simulink model "test_pos_ctrl_target"  (R2014a)
settings: Solver=ode5  StartTime=0.0  StopTime=inf  FixedStep=basic_time_step  RelTol=1e-3
values from neighbouring files (symbols this model uses):
  basic_time_step = 0.002    [init_pos_ctrl_target.m]
  g = 9.81    [init_pos_ctrl_target.m]
  kd = [2 0 0 ... (first row only)    [init_pos_ctrl_target.m]
  KDP = 11/5    (= 2.2)    [init_pos_ctrl_target.m]
  KDR = 11/5    (= 2.2)    [init_pos_ctrl_target.m]
  KDY = 11    [init_pos_ctrl_target.m]
  ki = 0*[.1 0 0 ... (first row only)    [init_pos_ctrl_target.m]
  kp = [1 0 0 ... (first row only)    [init_pos_ctrl_target.m]
  KPP = 30/5    (= 6)    [init_pos_ctrl_target.m]
  KPR = 30/5    (= 6)    [init_pos_ctrl_target.m]
  KPY = 30    [init_pos_ctrl_target.m]
  m0 = 1.3    [init_pos_ctrl_target.m]
  max_pitch = sin(15*pi/180)    [init_pos_ctrl_target.m]
  max_roll = sin(15*pi/180)    [init_pos_ctrl_target.m]
undefined symbols (not defined in the file or in its folder): DiscIntNeverNeededParam, IMU_time_step, n_robots, VICON_time_step
libraries: geometry_msgs x3, sensor_msgs x1, rt_sync x1
settings Model: Creator=prg  LastModifiedBy=fschiano
settings OptimizationCC: ExpressionDepthLimit=2147483647
settings DebuggingCC: UnderspecifiedInitializationDetection=Classic  StateNameClashWarn=warning

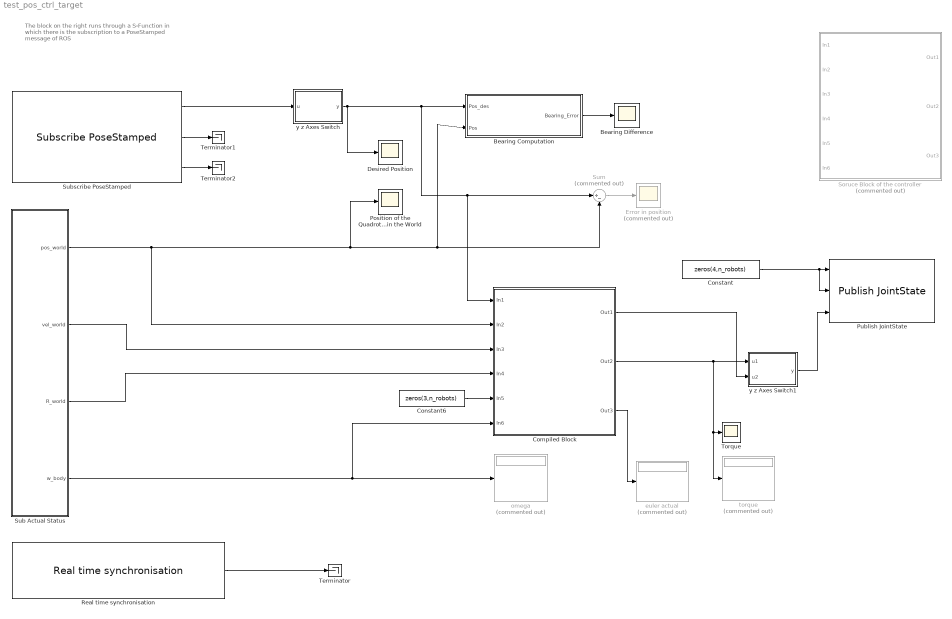
== system test_pos_ctrl_target ==
  note: The block on the right runs through a S-Function
      | in which there is the subscription to a PoseStamped
      | message of ROS
  Bearing Computation : Subsystem
  Bearing Difference : Scope
      settings: TimeRange=10000  YMin=-0.8  YMax=0.8  SaveName=ScopeData4
  Compiled Block : Subsystem
  Constant : Constant  Value=zeros(4,n_robots)  VectorParams1D=off
  Constant6 : Constant  Value=zeros(3,n_robots)
  Desired Position : Scope
      settings: TimeRange=10000  YMin=-4  YMax=7.5  SaveName=ScopeData3
  Error in position : Scope  Commented=on
      settings: TimeRange=10  YMin=-4  YMax=7.5
  "Position of the Quadrotor in the World " : Scope
      settings: TimeRange=10  YMin=-4  YMax=7.5  SaveName=ScopeData2
  Publish JointState : sensor_msgs/Publish JointState  stepTime=basic_time_step  topic_prefix='/command/quadrotor_'  list_of_robot_ids=char([0:n_robots-1])  topic_postfix=''  n_dofs=char(4)
  Real time synchronisation : rt_sync/Real time synchronisation  stepTime=basic_time_step  minShownDelay=0.5  ShowEveryNumCycles=1/basic_time_step  slowDownFactor=1
  Soruce Block of the controller : Subsystem  Commented=on
  Sub Actual Status : Subsystem
  Subscribe PoseStamped : geometry_msgs/Subscribe PoseStamped  stepTime=basic_time_step  topic_prefix='/vrep/Quadricopter_target_'  list_of_robot_ids=char([0:n_robots-1])  topic_postfix='/pose'
  Sum : Sum  Commented=on  Inputs=|+-
  Terminator : Terminator
  Terminator1 : Terminator
  Terminator2 : Terminator
  Torque : Scope
  euler actual : Display  Commented=on
  omega : Display  Commented=on
  "torque " : Display  Commented=on
  y z Axes Switch : MATLAB Function  TreatAsAtomicUnit=on
  y z Axes Switch1 : MATLAB Function  TreatAsAtomicUnit=on
  wires:
  Constant/1 -> Publish JointState/2, Publish JointState/1
  Sub Actual Status/4(w_body) -> Compiled Block/6(In6), omega/1
  Subscribe PoseStamped/1 -> y z Axes Switch/1(u)
  y z Axes Switch/1(y) -> Bearing Computation/1(Pos_des), Compiled Block/1(In1), Sum/1, Desired Position/1
  Sum/1 -> Error in position/1
  Real time synchronisation/1 -> Terminator/1
  Subscribe PoseStamped/2 -> Terminator1/1
  Subscribe PoseStamped/3 -> Terminator2/1
  Sub Actual Status/1(pos_world) -> Compiled Block/2(In2), Bearing Computation/2(Pos), Sum/2, "Position of the Quadrotor in the World "/1
  y z Axes Switch1/1(y) -> Publish JointState/3
  Compiled Block/2(Out2) -> "torque "/1, Torque/1, y z Axes Switch1/1(u1)
  Sub Actual Status/2(vel_world) -> Compiled Block/3(In3)
  Sub Actual Status/3("R_world ") -> Compiled Block/4(In4)
  Constant6/1 -> Compiled Block/5(In5)
  Compiled Block/1(Out1) -> y z Axes Switch1/2(u2)
  Compiled Block/3(Out3) -> euler actual/1
  Bearing Computation/1(Bearing_Error) -> Bearing Difference/1

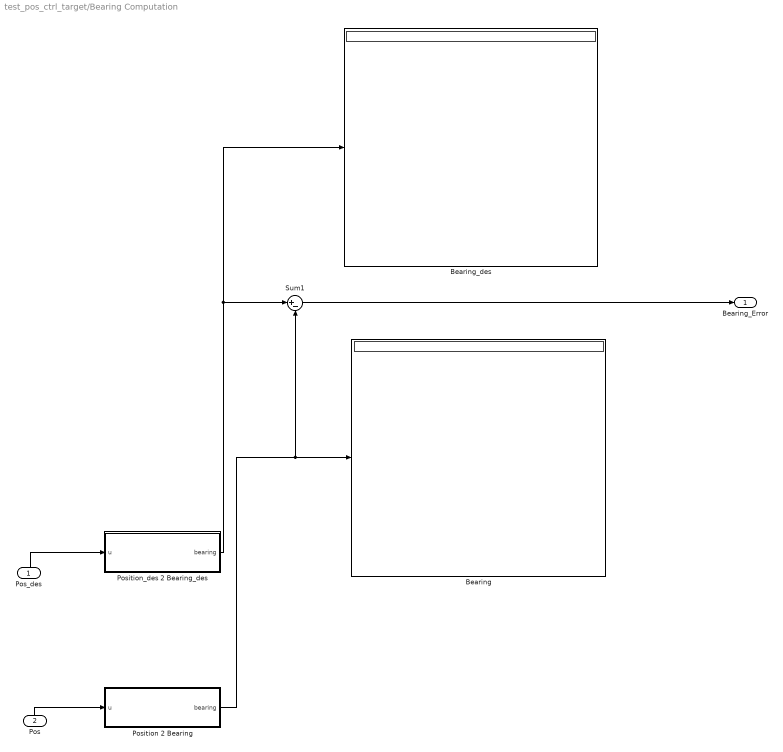
== system test_pos_ctrl_target/Bearing Computation ==
  Pos_des : Inport
  Pos : Inport  Port=2
  Bearing : Display
  "Bearing_des " : Display
  Position 2 Bearing : MATLAB Function  TreatAsAtomicUnit=on
  "Position_des 2 Bearing_des " : MATLAB Function  TreatAsAtomicUnit=on
  Sum1 : Sum  Inputs=|+-
  Bearing_Error : Outport
  wires:
  Pos/1 -> Position 2 Bearing/1(u)
  Pos_des/1 -> "Position_des 2 Bearing_des "/1(u)
  Position 2 Bearing/1(bearing) -> Bearing/1, Sum1/2
  Sum1/1 -> Bearing_Error/1
  "Position_des 2 Bearing_des "/1(bearing) -> Sum1/1, "Bearing_des "/1

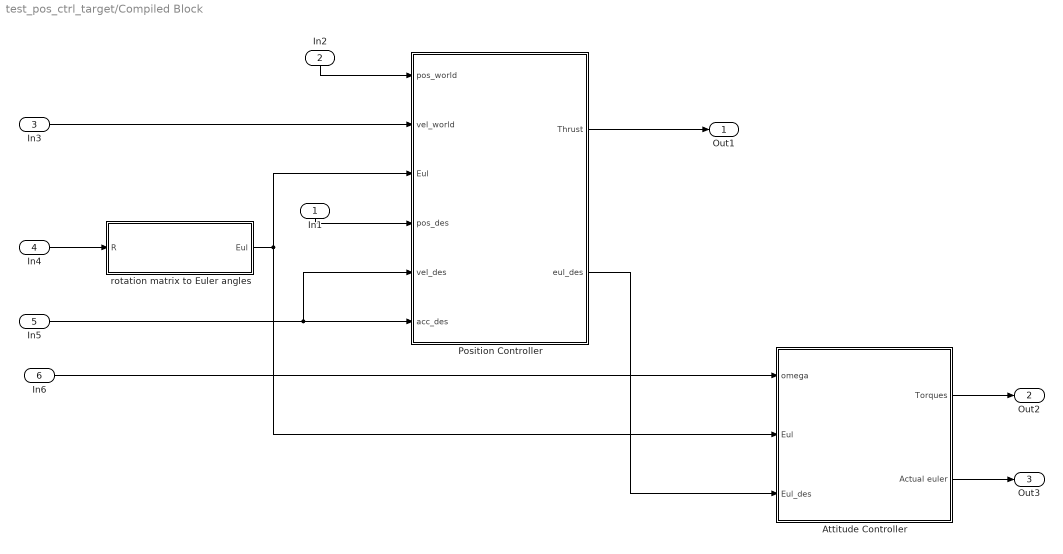
== system test_pos_ctrl_target/Compiled Block ==
  In1 : Inport
  In2 : Inport  Port=2
  In3 : Inport  Port=3
  In4 : Inport  Port=4
  In5 : Inport  Port=5
  In6 : Inport  Port=6
  Attitude Controller : Subsystem  SystemSampleTime=IMU_time_step
  Position Controller : Subsystem  SystemSampleTime=VICON_time_step
  rotation matrix to Euler angles : MATLAB Function  TreatAsAtomicUnit=on
  Out1 : Outport
  Out2 : Outport  Port=2
  Out3 : Outport  Port=3
  wires:
  In4/1 -> rotation matrix to Euler angles/1(R)
  rotation matrix to Euler angles/1(Eul) -> Attitude Controller/2(Eul), Position Controller/3(Eul)
  Attitude Controller/1(Torques) -> Out2/1
  In3/1 -> Position Controller/2(vel_world)
  In2/1 -> Position Controller/1(pos_world)
  Attitude Controller/2(Actual euler) -> Out3/1
  In1/1 -> Position Controller/4(pos_des)
  Position Controller/1(Thrust) -> Out1/1
  Position Controller/2(eul_des) -> Attitude Controller/3(Eul_des)
  In6/1 -> Attitude Controller/1(omega)
  In5/1 -> Position Controller/5(vel_des), Position Controller/6(acc_des)

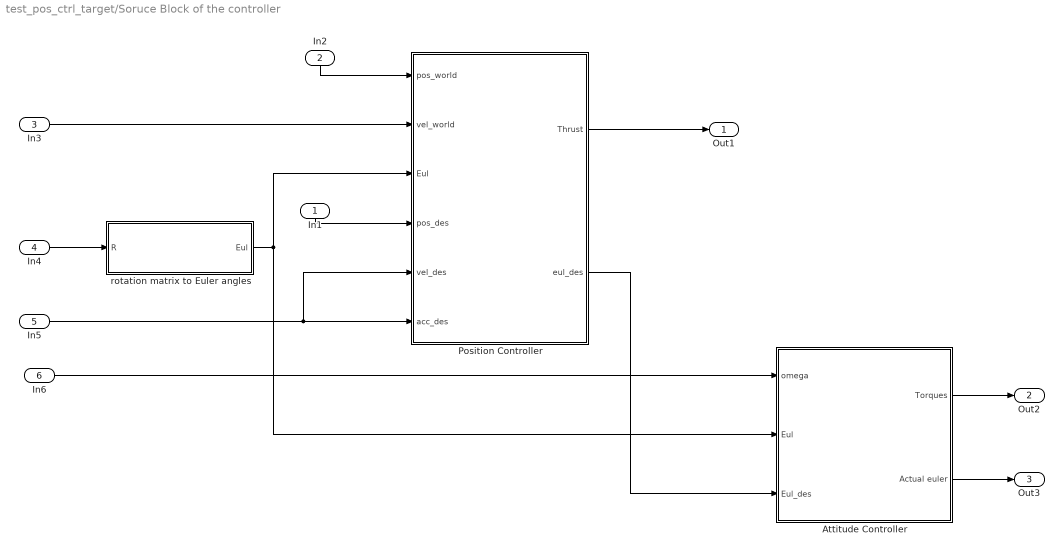
== system test_pos_ctrl_target/Soruce Block of the controller ==
  In1 : Inport
  In2 : Inport  Port=2
  In3 : Inport  Port=3
  In4 : Inport  Port=4
  In5 : Inport  Port=5
  In6 : Inport  Port=6
  Attitude Controller : Subsystem  SystemSampleTime=IMU_time_step
  Position Controller : Subsystem  SystemSampleTime=VICON_time_step
  rotation matrix to Euler angles : MATLAB Function  TreatAsAtomicUnit=on
  Out1 : Outport
  Out2 : Outport  Port=2
  Out3 : Outport  Port=3
  wires:
  In4/1 -> rotation matrix to Euler angles/1(R)
  rotation matrix to Euler angles/1(Eul) -> Attitude Controller/2(Eul), Position Controller/3(Eul)
  Attitude Controller/1(Torques) -> Out2/1
  In3/1 -> Position Controller/2(vel_world)
  In2/1 -> Position Controller/1(pos_world)
  Attitude Controller/2(Actual euler) -> Out3/1
  In1/1 -> Position Controller/4(pos_des)
  Position Controller/1(Thrust) -> Out1/1
  Position Controller/2(eul_des) -> Attitude Controller/3(Eul_des)
  In6/1 -> Attitude Controller/1(omega)
  In5/1 -> Position Controller/5(vel_des), Position Controller/6(acc_des)

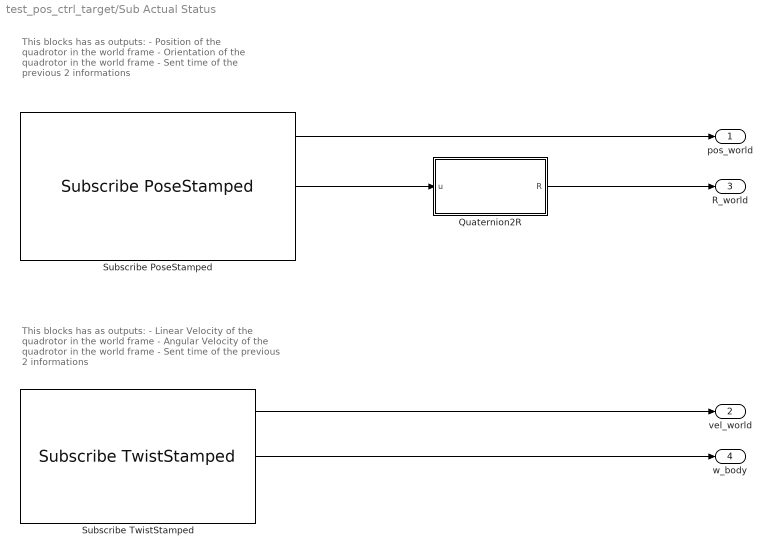
== system test_pos_ctrl_target/Sub Actual Status ==
  note: This blocks has as outputs:
      | - Linear Velocity of the quadrotor in the world frame
      | - Angular Velocity of the quadrotor in the world frame
      | - Sent time of the previous 2 informations
  note: This blocks has as outputs:
      | - Position of the quadrotor in the world frame
      | - Orientation of the quadrotor in the world frame
      | - Sent time of the previous 2 informations
  Quaternion2R : MATLAB Function  TreatAsAtomicUnit=on
  Subscribe PoseStamped : geometry_msgs/Subscribe PoseStamped  stepTime=basic_time_step  topic_prefix='/vrep/pose/quadrotor_'  list_of_robot_ids=char([0:n_robots-1])  topic_postfix=''
  Subscribe TwistStamped : geometry_msgs/Subscribe TwistStamped  stepTime=basic_time_step  topic_prefix='/vrep/twist/quadrotor_'  list_of_robot_ids=char([0:n_robots-1])  topic_postfix=''
  pos_world : Outport
  vel_world : Outport  Port=2
  "R_world " : Outport  Port=3
  w_body : Outport  Port=4
  wires:
  Subscribe PoseStamped/1 -> pos_world/1
  Subscribe PoseStamped/2 -> Quaternion2R/1(u)
  Quaternion2R/1(R) -> "R_world "/1
  Subscribe TwistStamped/1 -> vel_world/1
  Subscribe TwistStamped/2 -> w_body/1

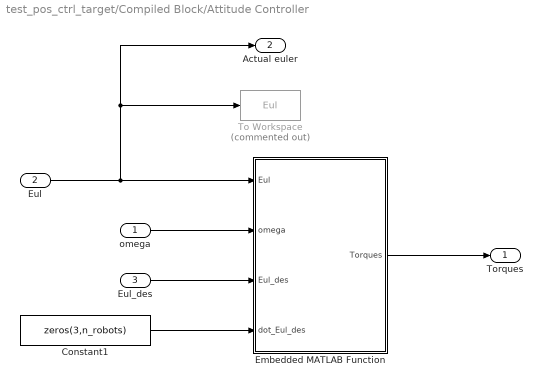
== system test_pos_ctrl_target/Compiled Block/Attitude Controller ==
  omega : Inport
  Eul : Inport  Port=2
  Eul_des : Inport  Port=3
  Constant1 : Constant  Value=zeros(3,n_robots)
  Embedded MATLAB Function : MATLAB Function  TreatAsAtomicUnit=on
  To Workspace : ToWorkspace  Commented=on  VariableName=Eul  SaveFormat=Structure With Time  SampleTime=-1
  Torques : Outport
  Actual euler : Outport  Port=2
  wires:
  Eul/1 -> Embedded MATLAB Function/1(Eul), Actual euler/1, To Workspace/1
  omega/1 -> Embedded MATLAB Function/2(omega)
  Eul_des/1 -> Embedded MATLAB Function/3(Eul_des)
  Embedded MATLAB Function/1(Torques) -> Torques/1
  Constant1/1 -> Embedded MATLAB Function/4(dot_Eul_des)

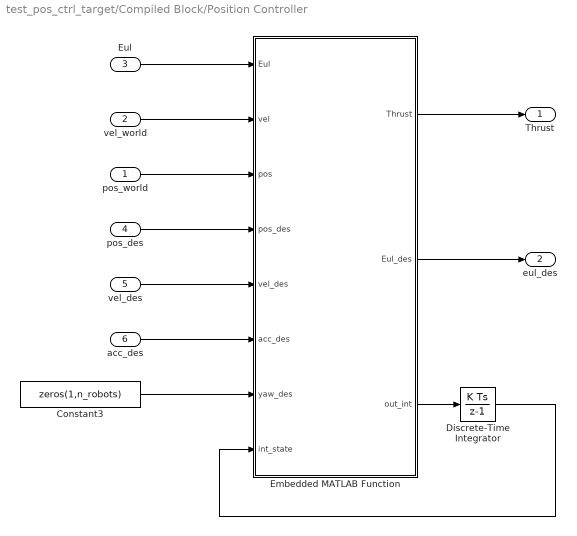
== system test_pos_ctrl_target/Compiled Block/Position Controller ==
  pos_world : Inport
  vel_world : Inport  Port=2
  Eul : Inport  Port=3
  pos_des : Inport  Port=4
  vel_des : Inport  Port=5
  acc_des : Inport  Port=6
  Constant3 : Constant  Value=zeros(1,n_robots)
  Discrete-Time Integrator : DiscreteIntegrator  InitialCondition=zeros(3,n_robots)  SampleTime=-1  OutDataTypeStr=Inherit: Inherit via back propagation  ICPrevOutput=DiscIntNeverNeededParam  ICPrevScaledInput=DiscIntNeverNeededParam
  Embedded MATLAB Function : MATLAB Function  TreatAsAtomicUnit=on
  Thrust : Outport
  eul_des : Outport  Port=2
  wires:
  Eul/1 -> Embedded MATLAB Function/1(Eul)
  vel_world/1 -> Embedded MATLAB Function/2(vel)
  pos_world/1 -> Embedded MATLAB Function/3(pos)
  Embedded MATLAB Function/1(Thrust) -> Thrust/1
  pos_des/1 -> Embedded MATLAB Function/4(pos_des)
  vel_des/1 -> Embedded MATLAB Function/5(vel_des)
  acc_des/1 -> Embedded MATLAB Function/6(acc_des)
  Constant3/1 -> Embedded MATLAB Function/7(yaw_des)
  Embedded MATLAB Function/3(out_int) -> Discrete-Time Integrator/1
  Discrete-Time Integrator/1 -> Embedded MATLAB Function/8(int_state)
  Embedded MATLAB Function/2(Eul_des) -> eul_des/1

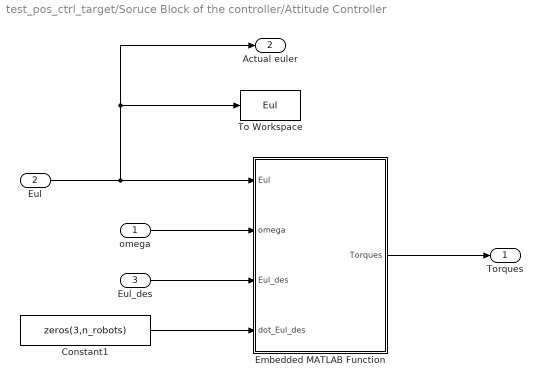
== system test_pos_ctrl_target/Soruce Block of the controller/Attitude Controller ==
  omega : Inport
  Eul : Inport  Port=2
  Eul_des : Inport  Port=3
  Constant1 : Constant  Value=zeros(3,n_robots)
  Embedded MATLAB Function : MATLAB Function  TreatAsAtomicUnit=on
  To Workspace : ToWorkspace  VariableName=Eul  SaveFormat=Structure With Time  SampleTime=-1
  Torques : Outport
  Actual euler : Outport  Port=2
  wires:
  Eul/1 -> Embedded MATLAB Function/1(Eul), Actual euler/1, To Workspace/1
  omega/1 -> Embedded MATLAB Function/2(omega)
  Eul_des/1 -> Embedded MATLAB Function/3(Eul_des)
  Embedded MATLAB Function/1(Torques) -> Torques/1
  Constant1/1 -> Embedded MATLAB Function/4(dot_Eul_des)

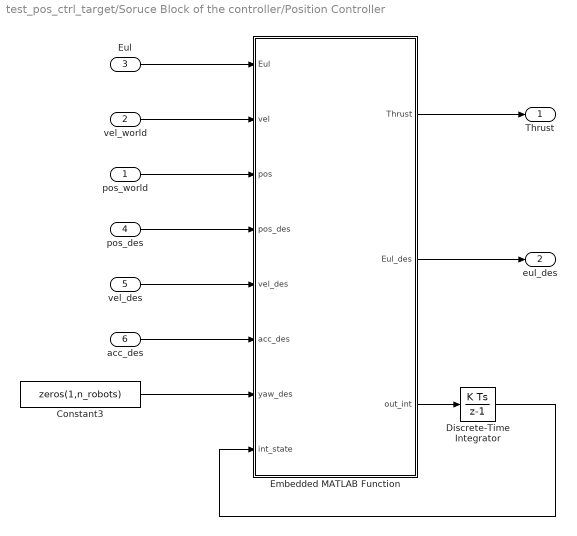
== system test_pos_ctrl_target/Soruce Block of the controller/Position Controller ==
  pos_world : Inport
  vel_world : Inport  Port=2
  Eul : Inport  Port=3
  pos_des : Inport  Port=4
  vel_des : Inport  Port=5
  acc_des : Inport  Port=6
  Constant3 : Constant  Value=zeros(1,n_robots)
  Discrete-Time Integrator : DiscreteIntegrator  InitialCondition=zeros(3,n_robots)  SampleTime=-1  OutDataTypeStr=Inherit: Inherit via back propagation  ICPrevOutput=DiscIntNeverNeededParam  ICPrevScaledInput=DiscIntNeverNeededParam
  Embedded MATLAB Function : MATLAB Function  TreatAsAtomicUnit=on
  Thrust : Outport
  eul_des : Outport  Port=2
  wires:
  Eul/1 -> Embedded MATLAB Function/1(Eul)
  vel_world/1 -> Embedded MATLAB Function/2(vel)
  pos_world/1 -> Embedded MATLAB Function/3(pos)
  Embedded MATLAB Function/1(Thrust) -> Thrust/1
  pos_des/1 -> Embedded MATLAB Function/4(pos_des)
  vel_des/1 -> Embedded MATLAB Function/5(vel_des)
  acc_des/1 -> Embedded MATLAB Function/6(acc_des)
  Constant3/1 -> Embedded MATLAB Function/7(yaw_des)
  Embedded MATLAB Function/3(out_int) -> Discrete-Time Integrator/1
  Discrete-Time Integrator/1 -> Embedded MATLAB Function/8(int_state)
  Embedded MATLAB Function/2(Eul_des) -> eul_des/1

== matlab function test_pos_ctrl_target/Soruce Block of the controller/Attitude Controller/Embedded MATLAB Function ==
  data: Eul input size=3,n_robots; Torques output size=3,n_robots; omega input size=3,n_robots; Eul_des input size=3,n_robots; dot_Eul_des input size=3,n_robots; KDR parameter; KPR parameter; KDP parameter; KPP parameter; KDY parameter; KPY parameter; n_robots parameter
% OLD FUNCTION (without parametrization for n_robots)
function Torques  = fcn(Eul, omega, Eul_des, dot_Eul_des, KDR, KPR, KDP, KPP, KDY, KPY, n_robots)
% This block supports the Embedded MATLAB subset.
% See the help menu for details.

% p = angles(2);
% r = angles(1);
% y=angles(3);
%
% T = [1      tan(p)*sin(r) tan(p)*cos(r);
%     0       cos(r)  -sin(r);
%     0       sin(r)/cos(p)   cos(r)/cos(p)];
%
% dot_ang = T*omega;
% dot_r=dot_ang(1);
% dot_p = dot_ang(2);
%
% T_dot = [0  tan(p)*cos(r)*dot_r+(sin(r)+tan(p)^2*sin(r))*dot_p -tan(p)*sin(r)*dot_r+(cos(r)+tan(p)^2*cos(r))*dot_p;
%          0  -sin(r)*dot_r   -cos(r)*dot_r;
%          0  cos(r)/cos(p)*dot_r+sin(r)*sin(p)/cos(p)^2*dot_p    -sin(r)/cos(p)*dot_r+cos(r)*sin(p)/cos(p)^2*dot_p];
%
%
% k_d = 11;
% k_p = 30;
% ang_vel_des = [0 0 yaw_dot_des]';
%
%
% if(yaw_des - angles(3) > pi)
%     angles(3) = angles(3)+2*pi;
% elseif (yaw_des - angles(3) < -pi)
%     angles(3) = angles(3)-2*pi;
% end
%
% ang_des = [roll_des pitch_des yaw_des]';
% U = I*inv(T)*(k_d*(ang_vel_des-dot_ang)+k_p*(ang_des - angles)-T_dot*omega)+cross(omega, I*omega);
% r_c = U(1);
% p_c = U(2);
% y_c = U(3);

Torques=[zeros(1,n_robots);zeros(1,n_robots);zeros(1,n_robots)];

% Extract Roll pitch and yaw angles w.r.t. the i-th robot
r = reshape(Eul(1,:),[1,1,n_robots]);
p = reshape(Eul(2,:),[1,1,n_robots]);
y = reshape(Eul(3,:),[1,1,n_robots]);

T = [ones(1,1,n_robots)       tan(p).*sin(r)  tan(p).*cos(r);
     zeros(1,1,n_robots)      cos(r)         -sin(r);
     zeros(1,1,n_robots)      sin(r)./cos(p)  cos(r)./cos(p)];


% T=eye(3);

dot_Eul = zeros(3,n_robots);

for i=1:n_robots
    dot_Eul(:,i)=reshape(T(:,:,i),[3,3])*omega(:,i);
end

% dot_Eul = T*omega;

dot_r = dot_Eul(1,:);
dot_p = dot_Eul(2,:);
dot_y = dot_Eul(3,:);

% U=I*inv(T)*([ KDR * (0 - dot_r) + KPR * (roll_des - r); KDP * (0 - dot_p) + KPP * (pitch_des - p) ; KPY * (yaw_dot_des - dot_y) ]);

r = reshape(r,[1,n_robots]);
p = reshape(p,[1,n_robots]);
y = reshape(y,[1,n_robots]);

Torques(1,:) = KDR * (dot_Eul_des(1,:) - dot_r) + KPR * (Eul_des(1,:) - r);
Torques(2,:) = KDP * (dot_Eul_des(2,:) - dot_p) + KPP * (Eul_des(2,:) - p);
Torques(3,:) = KDY * (dot_Eul_des(3,:) - dot_y) + KPY * (Eul_des(3,:) - y);


% if abs(Torques(1)) > 0.02
%     Torques(1)= 0.02;
%
% end
%
%
% if abs(Torques(2)) > 0.02
%     Torques(2)= 0.02;
%
% end

== matlab function test_pos_ctrl_target/Sub Actual Status/Quaternion2R ==
  data: u input size=4,n_robots; R output size=n_robots,3,3; n_robots parameter
function R = fcn(u, n_robots)

w = u(1,:);
x = u(2,:);
y = u(3,:);
z = u(4,:);

n = sqrt(x.*x + y.*y + z.*z + w.*w);

x = x./n;
y = y./n;
z = z./n;
w = w./n;

Rxx = reshape(1 - 2*(y.^2 + z.^2),[1,1,n_robots]);
Rxy = reshape(2*(x.*y - z.*w),[1,1,n_robots]);
Rxz = reshape(2*(x.*z + y.*w),[1,1,n_robots]);

Ryx = reshape(2*(x.*y + z.*w),[1,1,n_robots]);
Ryy = reshape(1 - 2*(x.^2 + z.^2),[1,1,n_robots]);
Ryz = reshape(2*(y.*z - x.*w ),[1,1,n_robots]);

Rzx = reshape(2*(x.*z - y.*w ),[1,1,n_robots]);
Rzy = reshape(2*(y.*z + x.*w ),[1,1,n_robots]);
Rzz = reshape(1 - 2 *(x.^2 + y.^2),[1,1,n_robots]);

R_temp = [
    Rxx,    Rxy,    Rxz;
    Ryx,    Ryy,    Ryz;
    Rzx,    Rzy,    Rzz;];

% R_temp = [
%     Rxx,    Ryx,    Rzx;
%     Rxy,    Ryy,    Rzy;
%     Rxz,    Ryz,    Rzz;];

% for i=1:n_robots
%     R_temp(:,:,i)=R_temp(:,:,i)';
% end

R=reshape(R_temp,n_robots,3,3);
% R=rand(1,3,3);

% a = u( 1 );
% b = u( 2 );
% c = u( 3 );
% d = u( 4 );
%
%
%   R(1,1) = a*a+b*b-c*c-d*d;
%   R(1,2) = 2*b*c-2*a*d;
%   R(1,3) = 2*a*c+2*b*d;
%
%   R(2,1)   = 2*a*d+2*b*c;
%   R(2,2)  = a*a-b*b+c*c-d*d;
%   R(2,3)  = 2*c*d-2*a*b;
%
%   R(3,1)    = 2*b*d-2*a*c;
%   R(3,2)    = 2*a*b+2*c*d;
%   R(3,3)    = a*a-b*b-c*c+d*d;


% % VERSION WITH THE FOR CYCLE
%
%
% % u is the vector of the quaternions.
% % If there are 2 robots involved the u will look like this:
% % u=[w1 x1 y1 z1 w2 x2 y2 z2]'
%
% %#codegen
% assert(n_robots<40);
%
% % Initialization of the variables. If you remove this it won't work because
% % code generation doesn't support dynamic changing size variables.
% w=zeros(n_robots,1);
% x=zeros(n_robots,1);
% y=zeros(n_robots,1);
% z=zeros(n_robots,1);
% n=zeros(n_robots,1);
%
% Rxx=zeros(n_robots,1);
% Rxy=zeros(n_robots,1);
% Rxz=zeros(n_robots,1);
% Ryx=zeros(n_robots,1);
% Ryy=zeros(n_robots,1);
% Ryz=zeros(n_robots,1);
% Rzx=zeros(n_robots,1);
% Rzy=zeros(n_robots,1);
% Rzz=zeros(n_robots,1);
%
% R=zeros(3*n_robots,3);
%
% for i=0:n_robots-1
%
%     w(i+1) = u( 1+3*i );
%     x(i+1) = u( 2+3*i );
%     y(i+1) = u( 3+3*i );
%     z(i+1) = u( 4+3*i );
%
%     n(i+1) = sqrt(x(i+1)*x(i+1) + y(i+1)*y(i+1) + z(i+1)*z(i+1) + w(i+1)*w(i+1));
%
%     x(i+1) = x(i+1)/ n(i+1);
%     y(i+1) = y(i+1)/ n(i+1);
%     z(i+1) = z(i+1)/ n(i+1);
%     w(i+1) = w(i+1)/ n(i+1);
%
%     Rxx(i+1) = 1 - 2*(y(i+1)^2 + z(i+1)^2);
%     Rxy(i+1) = 2*(x(i+1)*y(i+1) - z(i+1)*w(i+1));
%     Rxz(i+1) = 2*(x(i+1)*z(i+1) + y(i+1)*w(i+1));
%
%     Ryx(i+1) = 2*(x(i+1)*y(i+1) + z(i+1)*w(i+1));
%     Ryy(i+1) = 1 - 2*(x(i+1)^2 + z(i+1)^2);
%     Ryz(i+1) = 2*(y(i+1)*z(i+1) - x(i+1)*w(i+1) );
%
%     Rzx(i+1) = 2*(x(i+1)*z(i+1) - y(i+1)*w(i+1) );
%     Rzy(i+1) = 2*(y(i+1)*z(i+1) + x(i+1)*w(i+1) );
%     Rzz(i+1) = 1 - 2 *(x(i+1)^2 + y(i+1)^2);
%
%     R((1+i*3):(3+i*3),:) = [
%         Rxx(i+1),    Rxy(i+1),    Rxz(i+1);
%         Ryx(i+1),    Ryy(i+1),    Ryz(i+1);
%         Rzx(i+1),    Rzy(i+1),    Rzz(i+1)];
%
%     %     R_vectorized=R(:);
% end

== matlab function test_pos_ctrl_target/Soruce Block of the controller/Position Controller/Embedded MATLAB Function ==
  data: Eul input size=3,n_robots; Thrust output size=1,n_robots; Eul_des output size=3,n_robots; vel input size=3,n_robots; pos input size=3,n_robots; pos_des input size=3,n_robots; vel_des input size=3,n_robots; acc_des input size=3,n_robots; yaw_des input size=1,n_robots; int_state input size=3,n_robots; m0 parameter; g parameter; out_int output size=3,n_robots; kd parameter; kp parameter; ki parameter; max_roll parameter; max_pitch parameter; n_robots parameter
% Before the function was like that:
% function [Thrust, roll_des, pitch_des, yaw_dot_des, out_int]  = fcn(Eul, vel, pos, pos_des, vel_des, acc_des, yaw_des, int_state, m0, g, kd, kp, ki, max_roll, max_pitch,n_robots)

% Now I fused 3 variables roll_des, pitch_des, yaw_dot_des into Eul_des
function [Thrust, Eul_des, out_int]  = fcn(Eul, vel, pos, pos_des, vel_des, acc_des, yaw_des, int_state, m0, g, kd, kp, ki, max_roll, max_pitch,n_robots)
% This block supports the Embedded MATLAB subset
% See the help menu for details.

% Definition of the variables. For code generation, the first appearance
% of a variable must establish its size. The first appearance of a variable
% cannot be subscripted.

% r=zeros(n_robots,1);
% p=zeros(n_robots,1);
% y=zeros(n_robots,1);

% Thrust=zeros(n_robots,1);
%
% ddpx=zeros(n_robots,1);
% ddpy=zeros(n_robots,1);
%
% ctrl_roll=zeros(n_robots,1);
% ctrl_pitch=zeros(n_robots,1);
%
% roll_des=zeros(n_robots,1);
% pitch_des=zeros(n_robots,1);
% yaw_dot_des=zeros(n_robots,1);

% Extract Roll pitch and yaw angles w.r.t. the i-th robot
r = Eul(1,:);
p = Eul(2,:);
y = Eul(3,:);

% term_1=m0./(cos(r).*cos(p));
% term_2=(-g + acc_des(3,:) + kd(3,3)*(vel_des(3,:)-vel(3,:)) + kp(3,3)*(pos_des(3,:)-pos(3,:)) + int_state(3,:));
% term_3=term_1*term_2;

% Compute the Thrust w.r.t. the i-th robot
Thrust=m0./(cos(r).*cos(p)).*(-g + acc_des(3,:) + kd(3,3)*(vel_des(3,:)-vel(3,:)) + kp(3,3)*(pos_des(3,:)-pos(3,:)) + int_state(3,:) );

out_int=ki*(pos_des-pos);

% Saturation of the Thrust

for i=1:n_robots
    if (Thrust(1,i)>-5)
        Thrust(1,i)=-5;
    end
end

% max_T=30;
%
% if abs(T(3))>max_T
%     T(3)=sign(T(3))*max_T;
% end

% Thrust needed to hover ???
for i=1:n_robots
    if (Thrust(1,i)<-2*m0*g+5)
        Thrust(1,i)=-2*m0*g+5;
    end
end

% roll_des=-m/T(3)*( acc_des(2) + kd*(vel_des(2) -vel(2)) + kp*(pos_des(2)-pos(2)) );
% pitch_des=m/T(3)*( acc_des(1) + kd*(vel_des(1) -vel(1)) + kp*(pos_des(1)-pos(1)) );

ddpx=kd(1,1)*(vel_des(1,:) -vel(1,:)) + kp(1,1)*(pos_des(1,:)-pos(1,:) + int_state(1,:) );
ddpy=kd(2,2)*(vel_des(2,:) -vel(2,:)) + kp(2,2)*(pos_des(2,:)-pos(2,:) + int_state(2,:) );

ctrl_roll=m0./Thrust.*( -sin(y).*ddpx+cos(y).*ddpy);

% Saturation of the roll_ctrl
for i=1:n_robots
    if abs(ctrl_roll(1,i))>max_roll
        ctrl_roll(1,i)=sign(ctrl_roll(1,i))*max_roll;
    end 
end

ctrl_pitch= m0./(Thrust.*cos(r)).*( cos(y).*ddpx+sin(y).*ddpy);

% Saturation of the pitch_ctrl
for i=1:n_robots
    if abs(ctrl_pitch(1,i))>max_pitch
        ctrl_pitch(1,i)=sign(ctrl_pitch(1,i))*max_pitch;
    end
end


roll_des = -asin( ctrl_roll );

pitch_des = asin(  ctrl_pitch );

yaw_dot_des = zeros(1,n_robots); % kp(3,3)*(yaw_des-y);

Eul_des=([roll_des;pitch_des; yaw_dot_des]);


%% OLD FUNCTION (not parametrized for n_robots)
% function [Thrust, roll_des, pitch_des, yaw_dot_des, out_int]  = fcn(Eul, vel, pos, pos_des, vel_des, acc_des, yaw_des, int_state, m0, g, kd, kp, ki, max_roll, max_pitch)
% % This block supports the Embedded MATLAB subset
% % See the help menu for details.
%
%
% r = Eul(1);
% p = Eul(2);
% y = Eul(3);
%
%
%
% Thrust=m0/(cos(r)*cos(p))*(-g + acc_des(3) + kd(3,3)*(vel_des(3) -vel(3)) + kp(3,3)*(pos_des(3)-pos(3)) + int_state(3) );
%
%
% out_int=ki*(pos_des-pos);
%
%
%
% % max_T=30;
% %
% % if abs(T(3))>max_T
% %     T(3)=sign(T(3))*max_T;
% % end
%
% if (Thrust>-5)
%     Thrust=-5;
% end
%
%
% if (Thrust<-2*m0*g+5)
%     Thrust=-2*m0*g+5;
% end
%
%
%
%
% % roll_des=-m/T(3)*( acc_des(2) + kd*(vel_des(2) -vel(2)) + kp*(pos_des(2)-pos(2)) );
% % pitch_des=m/T(3)*( acc_des(1) + kd*(vel_des(1) -vel(1)) + kp*(pos_des(1)-pos(1)) );
%
%
% ddpx=kd(1,1)*(vel_des(1) -vel(1)) + kp(1,1)*(pos_des(1)-pos(1) + int_state(1) );
% ddpy=kd(2,2)*(vel_des(2) -vel(2)) + kp(2,2)*(pos_des(2)-pos(2) + int_state(2) );
%
%
%
% ctrl_roll=m0/Thrust*( -sin(y)*ddpx+cos(y)*ddpy);
%
% if abs(ctrl_roll)>max_roll
%     ctrl_roll=sign(ctrl_roll)*max_roll;
% end
%
% ctrl_pitch= m0/(Thrust*cos(r))*( cos(y)*ddpx+sin(y)*ddpy);
%
%
% if abs(ctrl_pitch)>max_pitch
%     ctrl_pitch=sign(ctrl_pitch)*max_pitch;
% end
%
%
%
%
%
% roll_des = -asin( ctrl_roll );
%
% pitch_des = asin(  ctrl_pitch );
%
% yaw_dot_des = 0; % kp(3,3)*(yaw_des-y);

== matlab function test_pos_ctrl_target/Soruce Block of the controller/rotation matrix to Euler angles ==
  data: R input size=n_robots,3,3 [..10]; Eul output size=3,n_robots; n_robots parameter
function Eul = eulerangles(R, n_robots)
% This block supports an embeddable subset of the MATLAB language.
% See the help menu for details.

R=reshape(R,[3,3,n_robots]);

Roll = atan2(R(3,2,:),R(3,3,:));
Pitch = atan2(-R(3,1,:),sqrt(R(3,2,:).^2+R(3,3,:).^2));
Yaw = atan2(R(2,1,:),R(1,1,:));

% From the previous instructions if R is a 3D matrix of 3 x 3 x n_robots I
% will have Roll Pitch and Yaw which will be 3 3D matrix with dimensions 1
% x 1 x n_robots. For this reason I need a reshape which will give
% transform Roll, Pitch and Yaw in vectors with dimensions 1 x n_robots

Roll = reshape(Roll,1,n_robots);
Pitch = reshape(Pitch,1,n_robots);
Yaw = reshape(Yaw,1,n_robots);

% The following Eul variable will be a 3 x n_robots matrix
Eul = [Roll; Pitch; Yaw];


% function Eul = eulerangles(R,n_robots)
% % This block supports an embeddable subset of the MATLAB language.
% % See the help menu for details.
% 
% % R=reshape(R_vectorized,[3,3,n_robots]);
% 
% Roll=zeros(n_robots);
% Pitch=zeros(n_robots);
% Yaw=zeros(n_robots);
% Eul=zeros(n_robots,3);
% 
% for i=1:n_robots
%     
%     Roll(i) = atan2(R(3+(n_robots-1)*3,2,i),R(3+(n_robots-1)*3,3,i));
%     Pitch(i) = atan2(-R(3+(n_robots-1)*3,1,i),sqrt(R(3+(n_robots-1)*3,2,i)^2+R(3+(n_robots-1)*3,3,i)^2));
%     Yaw(i) = atan2(R(2+(n_robots-1)*3,1,i),R(1+(n_robots-1)*3,1,i));
%     
%     Eul(i) = [Roll(i) Pitch(i) Yaw(i)];
% end

== matlab function test_pos_ctrl_target/Compiled Block/Attitude Controller/Embedded MATLAB Function ==
  data: Eul input size=3,n_robots; Torques output size=3,n_robots; omega input size=3,n_robots; Eul_des input size=3,n_robots; dot_Eul_des input size=3,n_robots; KDR parameter; KPR parameter; KDP parameter; KPP parameter; KDY parameter; KPY parameter; n_robots parameter
% OLD FUNCTION (without parametrization for n_robots)
function Torques  = fcn(Eul, omega, Eul_des, dot_Eul_des, KDR, KPR, KDP, KPP, KDY, KPY, n_robots)
% This block supports the Embedded MATLAB subset.
% See the help menu for details.

% p = angles(2);
% r = angles(1);
% y=angles(3);
%
% T = [1      tan(p)*sin(r) tan(p)*cos(r);
%     0       cos(r)  -sin(r);
%     0       sin(r)/cos(p)   cos(r)/cos(p)];
%
% dot_ang = T*omega;
% dot_r=dot_ang(1);
% dot_p = dot_ang(2);
%
% T_dot = [0  tan(p)*cos(r)*dot_r+(sin(r)+tan(p)^2*sin(r))*dot_p -tan(p)*sin(r)*dot_r+(cos(r)+tan(p)^2*cos(r))*dot_p;
%          0  -sin(r)*dot_r   -cos(r)*dot_r;
%          0  cos(r)/cos(p)*dot_r+sin(r)*sin(p)/cos(p)^2*dot_p    -sin(r)/cos(p)*dot_r+cos(r)*sin(p)/cos(p)^2*dot_p];
%
%
% k_d = 11;
% k_p = 30;
% ang_vel_des = [0 0 yaw_dot_des]';
%
%
% if(yaw_des - angles(3) > pi)
%     angles(3) = angles(3)+2*pi;
% elseif (yaw_des - angles(3) < -pi)
%     angles(3) = angles(3)-2*pi;
% end
%
% ang_des = [roll_des pitch_des yaw_des]';
% U = I*inv(T)*(k_d*(ang_vel_des-dot_ang)+k_p*(ang_des - angles)-T_dot*omega)+cross(omega, I*omega);
% r_c = U(1);
% p_c = U(2);
% y_c = U(3);

Torques=[zeros(1,n_robots);zeros(1,n_robots);zeros(1,n_robots)];

% Extract Roll pitch and yaw angles w.r.t. the i-th robot
r = reshape(Eul(1,:),[1,1,n_robots]);
p = reshape(Eul(2,:),[1,1,n_robots]);
y = reshape(Eul(3,:),[1,1,n_robots]);

T = [ones(1,1,n_robots)       tan(p).*sin(r)  tan(p).*cos(r);
     zeros(1,1,n_robots)      cos(r)         -sin(r);
     zeros(1,1,n_robots)      sin(r)./cos(p)  cos(r)./cos(p)];


% T=eye(3);

dot_Eul = zeros(3,n_robots);

for i=1:n_robots
    dot_Eul(:,i)=reshape(T(:,:,i),[3,3])*omega(:,i);
end

% dot_Eul = T*omega;

dot_r = dot_Eul(1,:);
dot_p = dot_Eul(2,:);
dot_y = dot_Eul(3,:);

% U=I*inv(T)*([ KDR * (0 - dot_r) + KPR * (roll_des - r); KDP * (0 - dot_p) + KPP * (pitch_des - p) ; KPY * (yaw_dot_des - dot_y) ]);

r = reshape(r,[1,n_robots]);
p = reshape(p,[1,n_robots]);
y = reshape(y,[1,n_robots]);

Torques(1,:) = KDR * (dot_Eul_des(1,:) - dot_r) + KPR * (Eul_des(1,:) - r);
Torques(2,:) = KDP * (dot_Eul_des(2,:) - dot_p) + KPP * (Eul_des(2,:) - p);
Torques(3,:) = KDY * (dot_Eul_des(3,:) - dot_y) + KPY * (Eul_des(3,:) - y);


% if abs(Torques(1)) > 0.02
%     Torques(1)= 0.02;
%
% end
%
%
% if abs(Torques(2)) > 0.02
%     Torques(2)= 0.02;
%
% end

== matlab function test_pos_ctrl_target/y z Axes Switch ==
  data: u input size=3,n_robots; y output size=3,n_robots; n_robots parameter
function y = fcn(u, n_robots)

y=[u(1,:);-u(2,:);-u(3,:)];

end

== matlab function test_pos_ctrl_target/y z Axes Switch1 ==
  data: u1 input; u2 input; y output; n_robots parameter
function y = fcn(u1,u2, n_robots)

y=[u1;u2];

end

== matlab function test_pos_ctrl_target/Compiled Block/Position Controller/Embedded MATLAB Function ==
  data: Eul input size=3,n_robots; Thrust output size=1,n_robots; Eul_des output size=3,n_robots; vel input size=3,n_robots; pos input size=3,n_robots; pos_des input size=3,n_robots; vel_des input size=3,n_robots; acc_des input size=3,n_robots; yaw_des input size=1,n_robots; int_state input size=3,n_robots; m0 parameter; g parameter; out_int output size=3,n_robots; kd parameter; kp parameter; ki parameter; max_roll parameter; max_pitch parameter; n_robots parameter
% Before the function was like that:
% function [Thrust, roll_des, pitch_des, yaw_dot_des, out_int]  = fcn(Eul, vel, pos, pos_des, vel_des, acc_des, yaw_des, int_state, m0, g, kd, kp, ki, max_roll, max_pitch,n_robots)

% Now I fused 3 variables roll_des, pitch_des, yaw_dot_des into Eul_des
function [Thrust, Eul_des, out_int]  = fcn(Eul, vel, pos, pos_des, vel_des, acc_des, yaw_des, int_state, m0, g, kd, kp, ki, max_roll, max_pitch,n_robots)
% This block supports the Embedded MATLAB subset
% See the help menu for details.

% Definition of the variables. For code generation, the first appearance
% of a variable must establish its size. The first appearance of a variable
% cannot be subscripted.

% r=zeros(n_robots,1);
% p=zeros(n_robots,1);
% y=zeros(n_robots,1);

% Thrust=zeros(n_robots,1);
%
% ddpx=zeros(n_robots,1);
% ddpy=zeros(n_robots,1);
%
% ctrl_roll=zeros(n_robots,1);
% ctrl_pitch=zeros(n_robots,1);
%
% roll_des=zeros(n_robots,1);
% pitch_des=zeros(n_robots,1);
% yaw_dot_des=zeros(n_robots,1);

% Extract Roll pitch and yaw angles w.r.t. the i-th robot
r = Eul(1,:);
p = Eul(2,:);
y = Eul(3,:);

% term_1=m0./(cos(r).*cos(p));
% term_2=(-g + acc_des(3,:) + kd(3,3)*(vel_des(3,:)-vel(3,:)) + kp(3,3)*(pos_des(3,:)-pos(3,:)) + int_state(3,:));
% term_3=term_1*term_2;

% Compute the Thrust w.r.t. the i-th robot
Thrust=m0./(cos(r).*cos(p)).*(-g + acc_des(3,:) + kd(3,3)*(vel_des(3,:)-vel(3,:)) + kp(3,3)*(pos_des(3,:)-pos(3,:)) + int_state(3,:) );

out_int=ki*(pos_des-pos);

% Saturation of the Thrust

for i=1:n_robots
    if (Thrust(1,i)>-5)
        Thrust(1,i)=-5;
    end
end

% max_T=30;
%
% if abs(T(3))>max_T
%     T(3)=sign(T(3))*max_T;
% end

% Thrust needed to hover ???
for i=1:n_robots
    if (Thrust(1,i)<-2*m0*g+5)
        Thrust(1,i)=-2*m0*g+5;
    end
end

% roll_des=-m/T(3)*( acc_des(2) + kd*(vel_des(2) -vel(2)) + kp*(pos_des(2)-pos(2)) );
% pitch_des=m/T(3)*( acc_des(1) + kd*(vel_des(1) -vel(1)) + kp*(pos_des(1)-pos(1)) );

ddpx=kd(1,1)*(vel_des(1,:) -vel(1,:)) + kp(1,1)*(pos_des(1,:)-pos(1,:) + int_state(1,:) );
ddpy=kd(2,2)*(vel_des(2,:) -vel(2,:)) + kp(2,2)*(pos_des(2,:)-pos(2,:) + int_state(2,:) );

ctrl_roll=m0./Thrust.*( -sin(y).*ddpx+cos(y).*ddpy);

% Saturation of the roll_ctrl
for i=1:n_robots
    if abs(ctrl_roll(1,i))>max_roll
        ctrl_roll(1,i)=sign(ctrl_roll(1,i))*max_roll;
    end 
end

ctrl_pitch= m0./(Thrust.*cos(r)).*( cos(y).*ddpx+sin(y).*ddpy);

% Saturation of the pitch_ctrl
for i=1:n_robots
    if abs(ctrl_pitch(1,i))>max_pitch
        ctrl_pitch(1,i)=sign(ctrl_pitch(1,i))*max_pitch;
    end
end


roll_des = -asin( ctrl_roll );

pitch_des = asin(  ctrl_pitch );

yaw_dot_des = zeros(1,n_robots); % kp(3,3)*(yaw_des-y);

Eul_des=([roll_des;pitch_des; yaw_dot_des]);


%% OLD FUNCTION (not parametrized for n_robots)
% function [Thrust, roll_des, pitch_des, yaw_dot_des, out_int]  = fcn(Eul, vel, pos, pos_des, vel_des, acc_des, yaw_des, int_state, m0, g, kd, kp, ki, max_roll, max_pitch)
% % This block supports the Embedded MATLAB subset
% % See the help menu for details.
%
%
% r = Eul(1);
% p = Eul(2);
% y = Eul(3);
%
%
%
% Thrust=m0/(cos(r)*cos(p))*(-g + acc_des(3) + kd(3,3)*(vel_des(3) -vel(3)) + kp(3,3)*(pos_des(3)-pos(3)) + int_state(3) );
%
%
% out_int=ki*(pos_des-pos);
%
%
%
% % max_T=30;
% %
% % if abs(T(3))>max_T
% %     T(3)=sign(T(3))*max_T;
% % end
%
% if (Thrust>-5)
%     Thrust=-5;
% end
%
%
% if (Thrust<-2*m0*g+5)
%     Thrust=-2*m0*g+5;
% end
%
%
%
%
% % roll_des=-m/T(3)*( acc_des(2) + kd*(vel_des(2) -vel(2)) + kp*(pos_des(2)-pos(2)) );
% % pitch_des=m/T(3)*( acc_des(1) + kd*(vel_des(1) -vel(1)) + kp*(pos_des(1)-pos(1)) );
%
%
% ddpx=kd(1,1)*(vel_des(1) -vel(1)) + kp(1,1)*(pos_des(1)-pos(1) + int_state(1) );
% ddpy=kd(2,2)*(vel_des(2) -vel(2)) + kp(2,2)*(pos_des(2)-pos(2) + int_state(2) );
%
%
%
% ctrl_roll=m0/Thrust*( -sin(y)*ddpx+cos(y)*ddpy);
%
% if abs(ctrl_roll)>max_roll
%     ctrl_roll=sign(ctrl_roll)*max_roll;
% end
%
% ctrl_pitch= m0/(Thrust*cos(r))*( cos(y)*ddpx+sin(y)*ddpy);
%
%
% if abs(ctrl_pitch)>max_pitch
%     ctrl_pitch=sign(ctrl_pitch)*max_pitch;
% end
%
%
%
%
%
% roll_des = -asin( ctrl_roll );
%
% pitch_des = asin(  ctrl_pitch );
%
% yaw_dot_des = 0; % kp(3,3)*(yaw_des-y);

== matlab function test_pos_ctrl_target/Compiled Block/rotation matrix to Euler angles ==
  data: R input size=n_robots,3,3 [..10]; Eul output size=3,n_robots; n_robots parameter
function Eul = eulerangles(R, n_robots)
% This block supports an embeddable subset of the MATLAB language.
% See the help menu for details.

R=reshape(R,[3,3,n_robots]);

Roll = atan2(R(3,2,:),R(3,3,:));
Pitch = atan2(-R(3,1,:),sqrt(R(3,2,:).^2+R(3,3,:).^2));
Yaw = atan2(R(2,1,:),R(1,1,:));

% From the previous instructions if R is a 3D matrix of 3 x 3 x n_robots I
% will have Roll Pitch and Yaw which will be 3 3D matrix with dimensions 1
% x 1 x n_robots. For this reason I need a reshape which will give
% transform Roll, Pitch and Yaw in vectors with dimensions 1 x n_robots

Roll = reshape(Roll,1,n_robots);
Pitch = reshape(Pitch,1,n_robots);
Yaw = reshape(Yaw,1,n_robots);

% The following Eul variable will be a 3 x n_robots matrix
Eul = [Roll; Pitch; Yaw];


% function Eul = eulerangles(R,n_robots)
% % This block supports an embeddable subset of the MATLAB language.
% % See the help menu for details.
% 
% % R=reshape(R_vectorized,[3,3,n_robots]);
% 
% Roll=zeros(n_robots);
% Pitch=zeros(n_robots);
% Yaw=zeros(n_robots);
% Eul=zeros(n_robots,3);
% 
% for i=1:n_robots
%     
%     Roll(i) = atan2(R(3+(n_robots-1)*3,2,i),R(3+(n_robots-1)*3,3,i));
%     Pitch(i) = atan2(-R(3+(n_robots-1)*3,1,i),sqrt(R(3+(n_robots-1)*3,2,i)^2+R(3+(n_robots-1)*3,3,i)^2));
%     Yaw(i) = atan2(R(2+(n_robots-1)*3,1,i),R(1+(n_robots-1)*3,1,i));
%     
%     Eul(i) = [Roll(i) Pitch(i) Yaw(i)];
% end

== matlab function test_pos_ctrl_target/Bearing Computation/Position_des 2 Bearing_des  ==
  data: u input size=3,n_robots; bearing output size=3*n_robots,n_robots; n_robots parameter
function bearing = fcn(u, n_robots)

bearing = zeros(3*n_robots,n_robots);

% bearing12=(u(:,2)-u(:,1))/(norm(u(:,2)-u(:,1)));

for i=1:n_robots
    for j=1:n_robots
        if (j==i)
            bearing(i+2*(i-1):3*i,j)=0;
        else
            bearing(i+2*(i-1):3*i,j)=(u(:,j)-u(:,i))/(norm(u(:,j)-u(:,i)));
        end
    end
end

end

== matlab function test_pos_ctrl_target/Bearing Computation/Position 2 Bearing ==
  data: u input size=3,n_robots; bearing output size=3*n_robots,n_robots; n_robots parameter
function bearing = fcn(u, n_robots)

bearing = zeros(3*n_robots,n_robots);

% bearing12=(u(:,2)-u(:,1))/(norm(u(:,2)-u(:,1)));

for i=1:n_robots
    for j=1:n_robots
        if (j==i)
            bearing(i+2*(i-1):3*i,j)=0;
        else
            bearing(i+2*(i-1):3*i,j)=(u(:,j)-u(:,i))/(norm(u(:,j)-u(:,i)));
        end
    end
end

end
